simulink model "Lab4_2"  (R2025a)
settings: Solver=VariableStepAuto  StartTime=0.0  StopTime=30.0  RelTol=1e-3
settings Model: Creator=andrei  LastModifiedBy=andrei

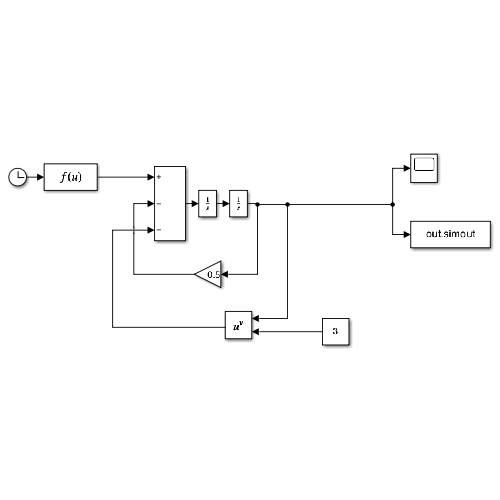
[thumbnail: Simulink's stored preview of the top-level diagram]
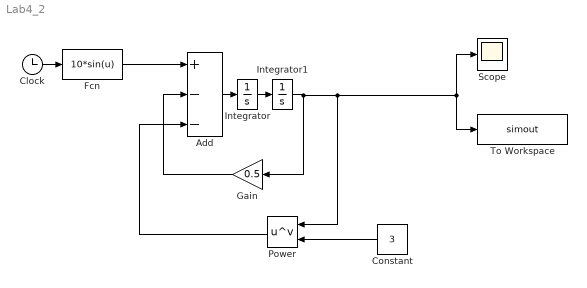
== system Lab4_2 ==
  Add : Sum  Inputs=+--
  Clock : Clock
  Constant : Constant  Value=3
  Fcn : Fcn  Expr=10*sin(u)
  Gain : Gain  Gain=0.5
  Integrator : Integrator
  Integrator1 : Integrator
  Power : Math  Operator=pow
  Scope : Scope
      settings: ActiveDisplayYMinimum=-9.1575824839286385E+9  ActiveDisplayYMaximum=1.3999722904070659E+9
  To Workspace : ToWorkspace  VariableName=simout  SampleTime=-1
  wires:
  Clock/1 -> Fcn/1
  Fcn/1 -> Add/1
  Add/1 -> Integrator/1
  Integrator/1 -> Integrator1/1
  Gain/1 -> Add/2
  Integrator1/1 -> Scope/1, To Workspace/1, Power/1, Gain/1
  Constant/1 -> Power/2
  Power/1 -> Add/3
